simulink model "lab6"  (R2021b)
settings: Solver=ode45  StartTime=0.0  StopTime=500  RelTol=1e-3  EnableMultiTasking=on
values from neighbouring files (symbols this model uses):
  ddMax = 3    [sysdata.m]
  deltaMax = 30    [sysdata.m]
  fConst = 0    [sysdata.m]
  K = 0.08    [lab2_otay.m]    (also in sysdata.m)
  Kaw = 8.1280    (= 8.128)    [lab6go.m]    (also in lab7go.m)
  Kc = 0.825    [sysdata.m]
  phiZad = 90    [sysdata.m]
  TI = 200    [sysdata.m]
  Toc = 5    [lab2_otay.m]    (also in sysdata.m)
  TR = 1    [lab2_otay.m]    (also in sysdata.m)
  Ts = 18.0    (= 18)    [lab2_otay.m]    (also in sysdata.m)
libraries: checkpacklib x1
settings Model: Creator=user  LastModifiedBy=Lapte
settings SolverCC: AlgebraicLoopSolver=TrustRegion
settings DataIOCC: LimitDataPoints=on  SaveFormat=Array  ReturnWorkspaceOutputs=off
settings OptimizationCC: LifeSpan=inf
settings DebuggingCC: SFUnexpectedBacktrackingDiag=warning  SFNoUnconditionalDefaultTransitionDiag=warning  SFExecutionAtInitializationDiag=none  SFMachineParentedDataDiag=warning  ArithmeticOperatorsInVariantConditions=warning
settings HardwareCC: ProdBitPerPointer=32  ProdBitPerSizeT=32  ProdBitPerPtrDiffT=32  ProdLargestAtomicFloat=None  ProdIntDivRoundTo=Undefined  ProdEndianess=Unspecified  ProdWordSize=32  ProdHWDeviceType=32-bit Generic
settings ModelReferenceCC: PropagateSignalLabelsOutOfModel=off
settings SFSimCC: SimUseLocalCustomCode=off  CustomCodeUndefinedFunction=UseInterfaceOnly
settings RTWCC: RTWUseLocalCustomCode=off
settings CodeAppCC: StateflowObjectComments=on
settings GRTTargetCC: TargetLangStandard=C89/C90 (ANSI)
settings ConfigComp: CovMetricSettings=dw  CovSaveCumulativeToWorkspaceVar=on  CovSaveSingleToWorkspaceVar=on  CovExternalEMLEnable=off  CovSFcnEnable=off

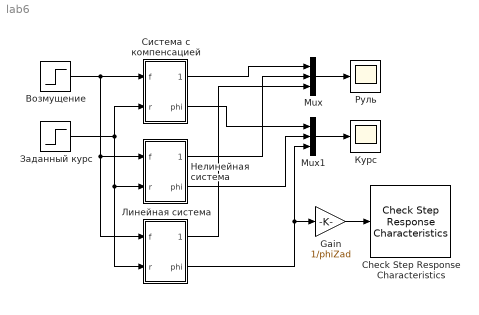
== system lab6 ==
  Check Step Response Characteristics : checkpacklib/Check Step Response  Characteristics  InstantiateOnLoad=on  enabled=on  stopWhenAssertionFail=off  export=off  ViewDlgPos=[]  OpenViewOnLoad=off  LaunchViewOnOpen=off  TimeUnits=seconds  EnableStepResponseBound=on  InitialValue=0  FinalValue=1  StepTime=0  RiseTime=65  PercentRise=82.3045267489712  SettlingTime=500  PercentSettling=3.90946502057614  PercentOvershoot=9.99999999999999  PercentUndershoot=1.02880658436214
      settings: SourceProductBaseCode=CT,ID,MT,SO
  Gain : Gain  Gain=1/phiZad
  Mux : Mux  Inputs=3
  Mux1 : Mux  Inputs=3
  Возмущение : Step  Time=0  After=fConst  SampleTime=0
  Заданный курс : Step  Time=0  After=phiZad  SampleTime=0
  Курс : Scope
  Линейная система : Subsystem
  Нелинейная система : Subsystem
  Руль : Scope
  Система с компенсацией : Subsystem
  wires:
  Возмущение/1 -> Линейная система/1(f), Нелинейная система/1(f), Система с компенсацией/1(f)
  Заданный курс/1 -> Линейная система/2(r), Нелинейная система/2(r), Система с компенсацией/2(r)
  Система с компенсацией/1(delta) -> Mux/1
  Система с компенсацией/2(phi) -> Mux1/1
  Нелинейная система/1(delta) -> Mux/2
  Нелинейная система/2(phi) -> Mux1/2
  Линейная система/1(delta) -> Mux/3
  Линейная система/2(phi) -> Gain/1, Mux1/3
  Mux/1 -> Руль/1
  Mux1/1 -> Курс/1
  Gain/1 -> Check Step Response Characteristics/1

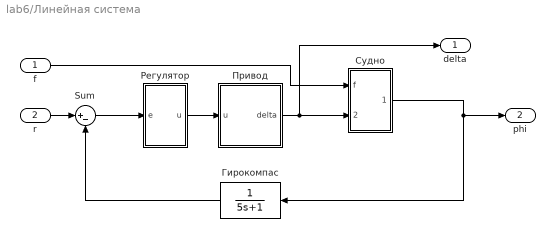
== system lab6/Линейная система ==
  f : Inport
  r : Inport  Port=2
  Sum : Sum  Inputs=|+-
  Гирокомпас : TransferFcn  Denominator=[5 1]
  Привод : Subsystem
  Регулятор : Subsystem
  Судно : Subsystem
  delta : Outport
  phi : Outport  Port=2
  wires:
  Регулятор/1(u) -> Привод/1(u)
  Судно/1(phi) -> phi/1, Гирокомпас/1
  Гирокомпас/1 -> Sum/2
  Sum/1 -> Регулятор/1(e)
  Привод/1(delta) -> delta/1, Судно/2(delta)
  r/1 -> Sum/1
  f/1 -> Судно/1(f)

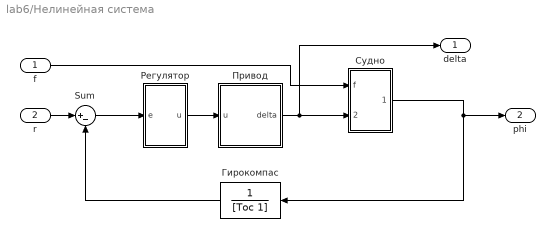
== system lab6/Нелинейная система ==
  f : Inport
  r : Inport  Port=2
  Sum : Sum  Inputs=|+-
  Гирокомпас : TransferFcn  Denominator=[Toc 1]
  Привод : Subsystem
  Регулятор : Subsystem
  Судно : Subsystem
  delta : Outport
  phi : Outport  Port=2
  wires:
  f/1 -> Судно/1(f)
  r/1 -> Sum/1
  Привод/1(delta) -> Судно/2(delta), delta/1
  Sum/1 -> Регулятор/1(e)
  Гирокомпас/1 -> Sum/2
  Судно/1(phi) -> Гирокомпас/1, phi/1
  Регулятор/1(u) -> Привод/1(u)

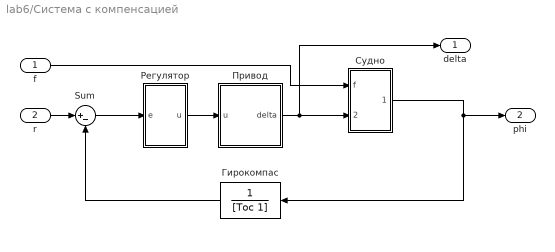
== system lab6/Система с компенсацией ==
  f : Inport
  r : Inport  Port=2
  Sum : Sum  Inputs=|+-
  Гирокомпас : TransferFcn  Denominator=[Toc 1]
  Привод : Subsystem
  Регулятор : Subsystem
  Судно : Subsystem
  delta : Outport
  phi : Outport  Port=2
  wires:
  f/1 -> Судно/1(f)
  r/1 -> Sum/1
  Привод/1(delta) -> Судно/2(delta), delta/1
  Sum/1 -> Регулятор/1(e)
  Гирокомпас/1 -> Sum/2
  Судно/1(phi) -> Гирокомпас/1, phi/1
  Регулятор/1(u) -> Привод/1(u)

== system lab6/Линейная система/Привод ==
  u : Inport
  Привод : TransferFcn  Denominator=[1 1]
  delta : Outport
  wires:
  Привод/1 -> delta/1
  u/1 -> Привод/1

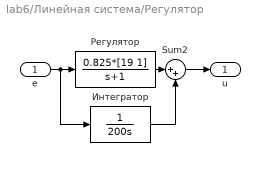
== system lab6/Линейная система/Регулятор ==
  e : Inport
  Sum2 : Sum  Inputs=|++
  Интегратор : TransferFcn  Denominator=[200 0]
  Регулятор : TransferFcn  Numerator=0.825*[19 1]  Denominator=[1 1]
  u : Outport
  wires:
  Интегратор/1 -> Sum2/2
  e/1 -> Интегратор/1, Регулятор/1
  Регулятор/1 -> Sum2/1
  Sum2/1 -> u/1

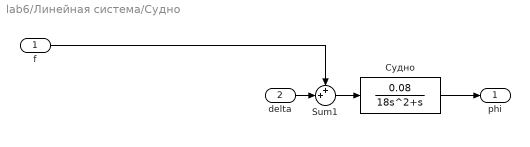
== system lab6/Линейная система/Судно ==
  f : Inport
  delta : Inport  Port=2
  Sum1 : Sum  Inputs=++|
  Судно : TransferFcn  Numerator=[0.08]  Denominator=[18 1 0]
  phi : Outport
  wires:
  delta/1 -> Sum1/2
  Sum1/1 -> Судно/1
  f/1 -> Sum1/1
  Судно/1 -> phi/1

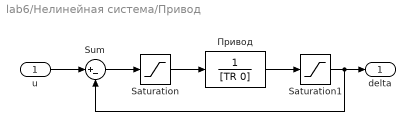
== system lab6/Нелинейная система/Привод ==
  u : Inport
  Saturation : Saturate  UpperLimit=TR*ddMax  LowerLimit=-TR*ddMax
  Saturation1 : Saturate  UpperLimit=deltaMax  LowerLimit=-deltaMax
  Sum : Sum  Inputs=|+-
  Привод : TransferFcn  Denominator=[TR 0]
  delta : Outport
  wires:
  Sum/1 -> Saturation/1
  u/1 -> Sum/1
  Saturation/1 -> Привод/1
  Привод/1 -> Saturation1/1
  Saturation1/1 -> delta/1, Sum/2

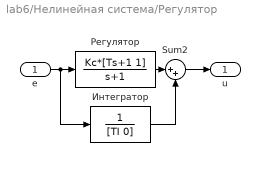
== system lab6/Нелинейная система/Регулятор ==
  e : Inport
  Sum2 : Sum  Inputs=|++
  Интегратор : TransferFcn  Denominator=[TI 0]
  Регулятор : TransferFcn  Numerator=Kc*[Ts+1 1]  Denominator=[1 1]
  u : Outport
  wires:
  Sum2/1 -> u/1
  Регулятор/1 -> Sum2/1
  e/1 -> Регулятор/1, Интегратор/1
  Интегратор/1 -> Sum2/2

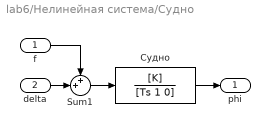
== system lab6/Нелинейная система/Судно ==
  f : Inport
  delta : Inport  Port=2
  Sum1 : Sum  Inputs=++|
  Судно : TransferFcn  Numerator=[K]  Denominator=[Ts 1 0]
  phi : Outport
  wires:
  Судно/1 -> phi/1
  f/1 -> Sum1/1
  Sum1/1 -> Судно/1
  delta/1 -> Sum1/2

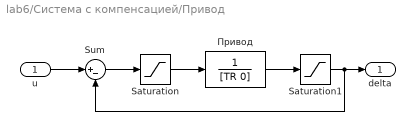
== system lab6/Система с компенсацией/Привод ==
  u : Inport
  Saturation : Saturate  UpperLimit=TR*ddMax  LowerLimit=-TR*ddMax
  Saturation1 : Saturate  UpperLimit=deltaMax  LowerLimit=-deltaMax
  Sum : Sum  Inputs=|+-
  Привод : TransferFcn  Denominator=[TR 0]
  delta : Outport
  wires:
  Sum/1 -> Saturation/1
  u/1 -> Sum/1
  Saturation/1 -> Привод/1
  Привод/1 -> Saturation1/1
  Saturation1/1 -> delta/1, Sum/2

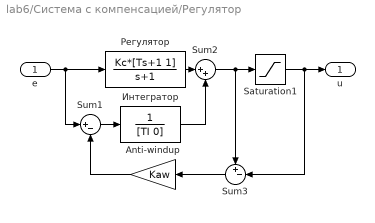
== system lab6/Система с компенсацией/Регулятор ==
  e : Inport
  Anti-windup : Gain  Gain=Kaw
  Saturation1 : Saturate  UpperLimit=deltaMax  LowerLimit=-deltaMax
  Sum1 : Sum  Inputs=|+-
  Sum2 : Sum  Inputs=|++
  Sum3 : Sum  Inputs=+-|
  Интегратор : TransferFcn  Denominator=[TI 0]
  Регулятор : TransferFcn  Numerator=Kc*[Ts+1 1]  Denominator=[1 1]
  u : Outport
  wires:
  Регулятор/1 -> Sum2/1
  e/1 -> Sum1/1, Регулятор/1
  Интегратор/1 -> Sum2/2
  Sum1/1 -> Интегратор/1
  Saturation1/1 -> u/1, Sum3/2
  Sum2/1 -> Sum3/1, Saturation1/1
  Sum3/1 -> Anti-windup/1
  Anti-windup/1 -> Sum1/2

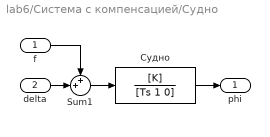
== system lab6/Система с компенсацией/Судно ==
  f : Inport
  delta : Inport  Port=2
  Sum1 : Sum  Inputs=++|
  Судно : TransferFcn  Numerator=[K]  Denominator=[Ts 1 0]
  phi : Outport
  wires:
  Судно/1 -> phi/1
  f/1 -> Sum1/1
  Sum1/1 -> Судно/1
  delta/1 -> Sum1/2
